simulink model "test_RC"  (R2017a)
settings: Solver=VariableStepAuto  StartTime=0.0  StopTime=5  FixedStep=1e-3  MaxStep=1e-3  RelTol=1e-3
libraries: slidercrank_basic_library_v1 x2, simulink x1, vrlib x1
settings Model: Creator=filip  LastModifiedBy=filip

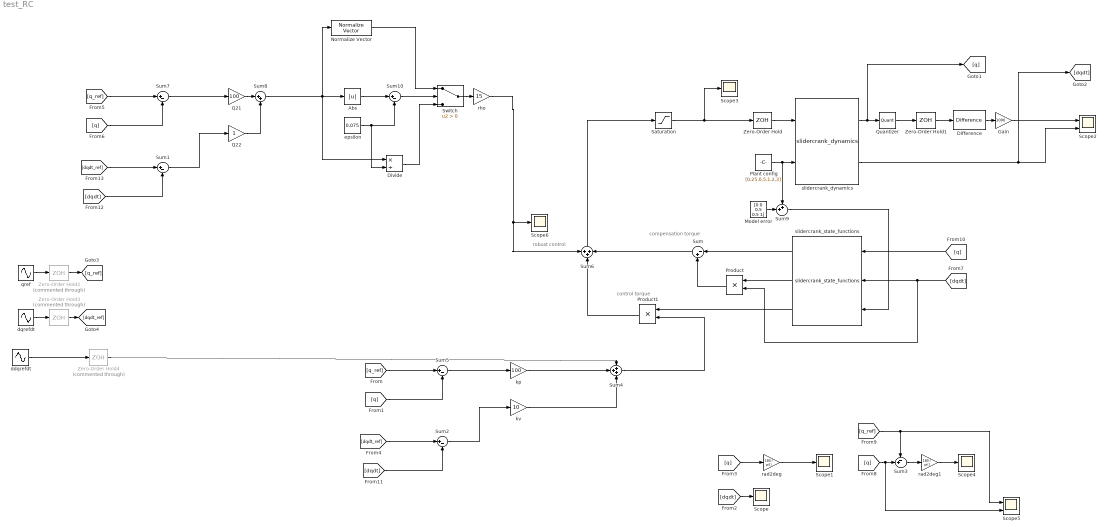
== system test_RC ==
  note: robust control
  note: compensation
      | torque
  note: control
      | torque
  Abs : Abs
  Difference : simulink/Discrete/Difference  ICPrevInput=0.0  OutMin=[]  OutMax=[]  OutDataType=fixdt(1, 16)  OutScaling=2^-10  DoSatur=off
  Divide : Product  Inputs=*/
  Gain : Gain  Gain=1000
  Model error : Constant  Value=[0 0 0.5 0.5 1]
  Normalize Vector : vrlib/Utilities/Normalize Vector  maxzero=0
      settings: SourceProductName=Simulink 3D Animation  SourceProductBaseCode=VR
  Plant config : Constant  Value=[0.25,0.5,1,2,3]
  Product : Product
  Product1 : Product
  Q21 : Gain  Gain=100
  Q22 : Gain
  Quantizer : Quantizer  QuantizationInterval=2*pi()/4096
  Saturation : Saturate  UpperLimit=45  LowerLimit=-45  LinearizeAsGain=off
  Scope{,1,3..4,6} (5 alike) : Scope
  Scope2 : Scope  NumInputPorts=2
  Scope5 : Scope  NumInputPorts=2
  Sum : Sum  Inputs=|-+
  Sum{1..2,5,7,10} (5 alike) : Sum  Inputs=|+-
  Sum3 : Sum  Inputs=-+|
  Sum4 : Sum  Inputs=+++
  Sum6 : Sum  Inputs=+++
  Sum8 : Sum  Inputs=|++
  Sum9 : Sum  Inputs=++|
  Switch : Switch  Criteria=u2 > Threshold
  Zero-Order Hold : ZeroOrderHold  SampleTime=1e-3
  Zero-Order Hold1 : ZeroOrderHold  SampleTime=1e-3
  Zero-Order Hold2 : ZeroOrderHold  Commented=through  SampleTime=1e-3
  Zero-Order Hold3 : ZeroOrderHold  Commented=through  SampleTime=1e-3
  Zero-Order Hold4 : ZeroOrderHold  Commented=through  SampleTime=1e-3
  ddqrefdt : Sin  Amplitude=-100  Frequency=10  SampleTime=0
  dqrefdt : Sin  Amplitude=10  Frequency=10  Phase=pi()/2*10/2  SampleTime=0
  epsilon : Constant  Value=0.075
  kp : Gain  Gain=100
  kv : Gain  Gain=10
  qref : Sin  Frequency=10  SampleTime=0
  rad2deg : Gain  Gain=180 / pi()
  rad2deg1 : Gain  Gain=180 / pi()
  rho : Gain  Gain=15
  slidercrank_dynamics : slidercrank_basic_library_v1/slidercrank_dynamics
  slidercrank_state_functions : slidercrank_basic_library_v1/slidercrank_state_functions
  wires:
  Plant config/1 -> Sum9/1, slidercrank_dynamics/2
  [dqdt] -> Scope/1
  [q] -> rad2deg/1
  rad2deg/1 -> Scope1/1
  ddqrefdt/1 -> Zero-Order Hold4/1
  [q] -> Scope5/2, Sum3/2
  Sum3/1 -> rad2deg1/1
  rad2deg1/1 -> Scope4/1
  [q_ref] -> Scope5/1, Sum3/1
  Sum9/1 -> slidercrank_state_functions/3
  [q] -> slidercrank_state_functions/1
  [dqdt] -> Product/2, slidercrank_state_functions/2
  slidercrank_state_functions/2 -> Product/1
  slidercrank_state_functions/1 -> Sum/1
  Product/1 -> Sum/2
  slidercrank_state_functions/3 -> Product1/1
  Sum4/1 -> Product1/2
  kp/1 -> Sum4/2
  kv/1 -> Sum4/3
  [dqdt_ref] -> Sum2/1
  [dqdt] -> Sum2/2
  Sum2/1 -> kv/1
  [q_ref] -> Sum5/1
  [q] -> Sum5/2
  Sum5/1 -> kp/1
  dqrefdt/1 -> Zero-Order Hold3/1
  qref/1 -> Zero-Order Hold2/1
  Zero-Order Hold/1 -> slidercrank_dynamics/1
  Sum6/1 -> Saturation/1
  slidercrank_dynamics/1 -> [q], Quantizer/1
  Zero-Order Hold1/1 -> Difference/1
  Quantizer/1 -> Zero-Order Hold1/1
  Difference/1 -> Gain/1
  Gain/1 -> Scope2/1
  Saturation/1 -> Scope3/1, Zero-Order Hold/1
  Zero-Order Hold2/1 -> [q_ref]
  Zero-Order Hold3/1 -> [dqdt_ref]
  Zero-Order Hold4/1 -> Sum4/1
  Product1/1 -> Sum6/2
  Sum/1 -> Sum6/3
  [q_ref] -> Sum7/1
  [dqdt] -> Sum1/2
  Sum7/1 -> Q21/1
  Sum1/1 -> Q22/1
  [dqdt_ref] -> Sum1/1
  [q] -> Sum7/2
  Q21/1 -> Sum8/1
  Q22/1 -> Sum8/2
  Model error/1 -> Sum9/2
  rho/1 -> Scope6/1, Sum6/1
  slidercrank_dynamics/2 -> [dqdt], Scope2/2
  Switch/1 -> rho/1
  Sum10/1 -> Switch/2
  Normalize Vector/1 -> Switch/1
  Sum8/1 -> Divide/1, Normalize Vector/1, Abs/1
  Abs/1 -> Sum10/1
  epsilon/1 -> Divide/2, Sum10/2
  Divide/1 -> Switch/3
